simulink library "lib_S7RRRRRRR1_kinematics"  (Simulink 8.5)
settings: Solver=ode45  StartTime=0.0  StopTime=10.0  RelTol=1e-3
undefined symbols (not defined in the file or in its folder): pkin
settings Model: Creator=schappler  LastModifiedBy=schappler

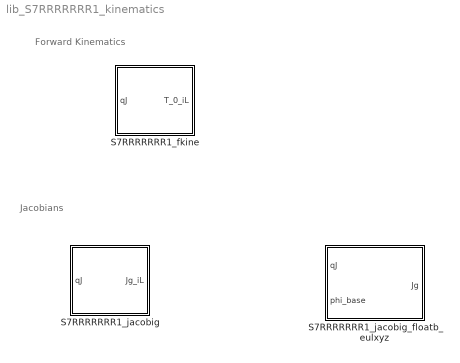
== system lib_S7RRRRRRR1_kinematics ==
  note: Jacobians
  note: Forward Kinematics
  S7RRRRRRR1_fkine : Subsystem  mask{pkin=pkin, iL=0}
      mask prompts: pkin "Kinematik-Parameter"; iL "Segment-Nummer (0=Basis)"
      mask init:
      | NQJ=7;
      mask Display:
      | text(0.5,0.8, 'fkine', 'horizontalAlignment', 'center');
      | text(0.5,0.2, sprintf('Link %d', iL), 'horizontalAlignment', 'center');
      | port_label('input', 1, 'qJ');
      | port_label('output', 1, sprintf('T_0_%d', iL));
  S7RRRRRRR1_jacobig : Subsystem  mask{pkin=pkin, iL=0, r_i_i_C=zeros(3,1)}
      mask prompts: pkin "Kinematik-Parameter"; iL "Segment-Nummer (0=Basis)"; r_i_i_C "Koordinaten zum betrachteten Punkt in Körper-KS: r_i_i_C"
      mask init:
      | NQJ=7;
      mask Display:
      | text(0.5,0.8, 'Jacobi (geom)\nfixed-base', 'horizontalAlignment', 'center');
      | text(0.5,0.2, sprintf('Link %d', iL), 'horizontalAlignment', 'center');
      | port_label('input', 1, 'qJ');
      | port_label('output', 1, sprintf('Jg_%d', iL));
  S7RRRRRRR1_jacobig_floatb_eulxyz : Subsystem  mask{pkin=pkin, iL=0, r_i_i_C=zeros(3,1)}
      mask prompts: pkin "Kinematik-Parameter"; iL "Segment-Nummer (0=Basis)"; r_i_i_C "Koordinaten zum betrachteten Punkt in Körper-KS: r_i_i_C"
      mask init:
      | NQJ=7;
      mask Display:
      | text(0.5,0.8, 'Jacobi (geom)\nfloating-base', 'horizontalAlignment', 'center');
      | text(0.5,0.2, sprintf('Link %d', iL), 'horizontalAlignment', 'center');
      | port_label('input', 1, 'q_J', 'interpreter', 'tex');
      | port_label('input', 2, '\phi_B', 'interpreter', 'tex');
      | port_label('output', 1, sprintf('J_{g,%d}', iL), 'interpreter', 'tex');

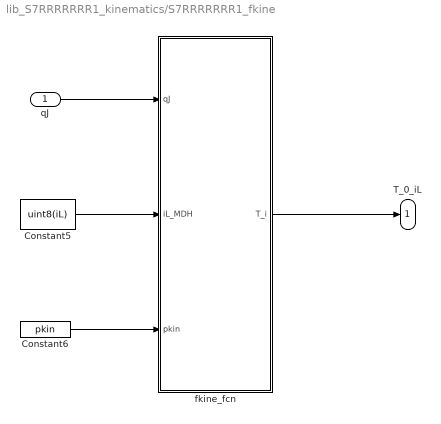
== system lib_S7RRRRRRR1_kinematics/S7RRRRRRR1_fkine ==
  qJ : Inport  PortDimensions=NQJ
  Constant5 : Constant  Value=uint8(iL)
  Constant6 : Constant  Value=pkin
  fkine_fcn : MATLAB Function  TreatAsAtomicUnit=on
  T_0_iL : Outport
  wires:
  fkine_fcn/1(T_i) -> T_0_iL/1
  Constant6/1 -> fkine_fcn/3(pkin)
  qJ/1 -> fkine_fcn/1(qJ)
  Constant5/1 -> fkine_fcn/2(iL_MDH)

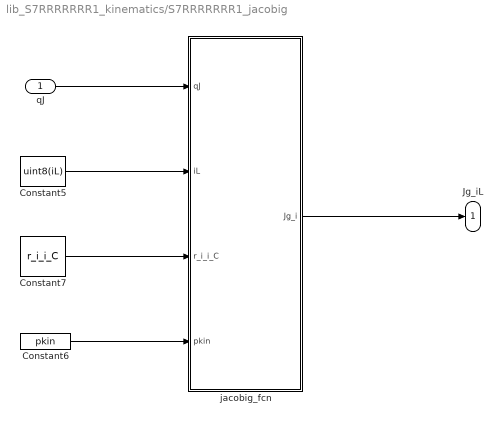
== system lib_S7RRRRRRR1_kinematics/S7RRRRRRR1_jacobig ==
  qJ : Inport  PortDimensions=NQJ
  Constant5 : Constant  Value=uint8(iL)
  Constant6 : Constant  Value=pkin
  Constant7 : Constant  Value=r_i_i_C
  jacobig_fcn : MATLAB Function  TreatAsAtomicUnit=on
  Jg_iL : Outport  PortDimensions=[6 NQJ]
      mask init:
      | NQJ=7;
  wires:
  jacobig_fcn/1(Jg_i) -> Jg_iL/1
  Constant6/1 -> jacobig_fcn/4(pkin)
  qJ/1 -> jacobig_fcn/1(qJ)
  Constant5/1 -> jacobig_fcn/2(iL)
  Constant7/1 -> jacobig_fcn/3(r_i_i_C)

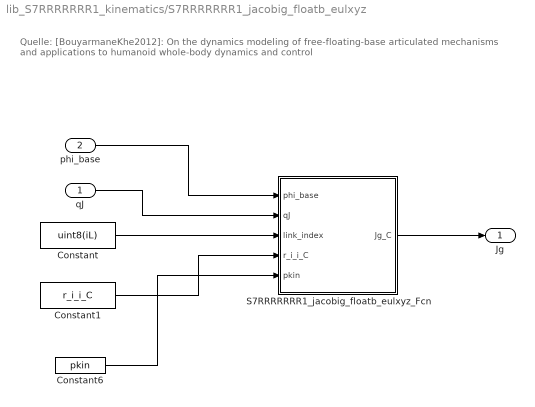
== system lib_S7RRRRRRR1_kinematics/S7RRRRRRR1_jacobig_floatb_eulxyz ==
  note: Quelle:
      | [BouyarmaneKhe2012]: On the dynamics modeling of free-floating-base articulated mechanisms and applications to humanoid whole-body dynamics and control
  qJ : Inport  PortDimensions=NQJ
  phi_base : Inport  Port=2  PortDimensions=3
  Constant : Constant  Value=uint8(iL)
  Constant1 : Constant  Value=r_i_i_C
  Constant6 : Constant  Value=pkin
  S7RRRRRRR1_jacobig_floatb_eulxyz_Fcn : MATLAB Function  TreatAsAtomicUnit=on
  Jg : Outport  PortDimensions=[6 (NQJ+6)]
  wires:
  phi_base/1 -> S7RRRRRRR1_jacobig_floatb_eulxyz_Fcn/1(phi_base)
  S7RRRRRRR1_jacobig_floatb_eulxyz_Fcn/1(Jg_C) -> Jg/1
  Constant/1 -> S7RRRRRRR1_jacobig_floatb_eulxyz_Fcn/3(link_index)
  Constant1/1 -> S7RRRRRRR1_jacobig_floatb_eulxyz_Fcn/4(r_i_i_C)
  qJ/1 -> S7RRRRRRR1_jacobig_floatb_eulxyz_Fcn/2(qJ)
  Constant6/1 -> S7RRRRRRR1_jacobig_floatb_eulxyz_Fcn/5(pkin)

== matlab function S7RRRRRRR1_jacobig/jacobig_fcn ==
  data: qJ input double; Jg_i output double; iL input double; r_i_i_C input double; pkin input double
function Jg_i = jacobig(qJ, iL, r_i_i_C, pkin)
%#codegen
% Segmentnummer wird in MDH-Notation übergeben (0=Basis).
Jg_i = S7RRRRRRR1_jacobig_sym_varpar(qJ, iL, r_i_i_C, pkin);

== matlab function S7RRRRRRR1_fkine/fkine_fcn ==
  data: qJ input double; T_i output double; iL_MDH input double; pkin input double
function T_i = fkine(qJ, iL_MDH, pkin)
%#codegen
T_c_mdh = S7RRRRRRR1_fkine_fixb_rotmat_mdh_sym_varpar(qJ, pkin);
% Segmentnummer wird in MDH-Notation übergeben (0=Basis). Die Matlab-Arrays
% fangen bei 1 an.
T_i = T_c_mdh(:,:,iL_MDH+1);

== matlab function S7RRRRRRR1_jacobig_floatb_eulxyz/S7RRRRRRR1_jacobig_floatb_eulxyz_Fcn ==
  data: phi_base input double; qJ input double; Jg_C output double; link_index input uint8 size=1; r_i_i_C input double; pkin input double
% Floating-Base Jacobimatrix zu beliebigen Punkten

function Jg_C = fcn(phi_base, qJ, link_index, r_i_i_C, pkin)
%% Init
%#codegen
% Segmentnummer wird in MDH-Notation übergeben (0=Basis).
Jg_C = S7RRRRRRR1_jacobig_mdh_eulxyz_sym(phi_base, qJ, link_index, r_i_i_C, pkin);
